simulink model "ModeAdjust"  (R2018b)
settings: Solver=FixedStepDiscrete  StartTime=0.0  StopTime=inf  FixedStep=0.01  RelTol=1e-3
undefined symbols (not defined in the file or in its folder): IfKeSMSbSeatMovBkRclnEnable_Val, IfKeSMSbSeatMovFrwdBkwdEnable_Val, IfKeSMSbSeatMovFtrstEnable_Val, IfKeSMSbSeatMovHdrstFrwdBkwdEnable_Val, IfKeSMSbSeatMovHdUpwdDnwdEnable_Val, IfKeSMSbSeatMovLgrstEnable_Val, IfKeSMSbSeatMovLtwdRtwdEnable_Val, IfVeSMSeStNumConfig, KeSMSbArmscreenMovEnable_Val, KeSMSbSeatMovLgrstExpdEnable_Val, KeSMSuFirstRwStBackPosDelta_Val, KeSMSuFirstRwStBackPosTolr_Val, KeSMSuFirstRwStCushFrntPosDelta_Val, KeSMSuFirstRwStCushFrntPosTolr_Val, KeSMSuFirstRwStCushRePosDelta_Val, KeSMSuFirstRwStCushRePosTolr_Val, KeSMSuFirstRwStFootrestPosDelta_Val, KeSMSuFirstRwStFootrestPosTolr_Val, KeSMSuFirstRwStFwdBkwdPosDelta_Val, KeSMSuFirstRwStFwdBkwdPosTolr_Val, KeSMSuMdMotFinshdTm_Val, KeSMSuMdRetryTm1_Val, KeSMSuModeReqDurgTm_Val, KeSMSuSecRwStArmTochPosDelta_Val, KeSMSuSecRwStArmTochPosTolr_Val, KeSMSuSecRwStBackPosDelta_Val, KeSMSuSecRwStBackPosTolr_Val, KeSMSuSecRwStFtrstUpwdDnwdPosDelta_Val, KeSMSuSecRwStFtrstUpwdDnwdPosTolr_Val, KeSMSuSecRwStFwdBkwdPosDelta_Val, KeSMSuSecRwStFwdBkwdPosTolr_Val, KeSMSuSecRwStHeadrestFwdBkwdPosDelta_Val, KeSMSuSecRwStHeadrestFwdBkwdPosTolr_Val, KeSMSuSecRwStHeadrestUpwdDwnwdPosDelta_Val, KeSMSuSecRwStHeadrestUpwdDwnwdPosTolr_Val, KeSMSuSecRwStLegrestInOutPosDelta_Val, KeSMSuSecRwStLegrestInOutPosTolr_Val, KeSMSuSecRwStLegrestUpwdDwnwdPosDelta_Val, KeSMSuSecRwStLegrestUpwdDwnwdPosTolr_Val, KeSMSuSecRwStLwdRwdPosDelta_Val, KeSMSuSecRwStLwdRwdPosTolr_Val, KeSMSuSecRwStVIPFtrstRefAngle_Val, KeSMSuThirdRwStFwdBkwdPosDelta_Val, KeSMSuThirdRwStFwdBkwdPosTolr_Val, KeSMSuThrdRwCushFoldPosDelta_Val, KeSMSuThrdRwCushFoldPosTolr_Val, KeSMSuThrdRwStBackPosDelta_Val, KeSMSuThrdRwStBackPosTolr_Val, KeSMSw4SLegrstCloseMdSecRwLtStFtrstUpwdDnwdPos_Val, KeSMSw4SLegrstCloseMdSecRwLtStFtrstUpwdDnwdPosMax_Val, KeSMSw4SLegrstCloseMdSecRwLtStFtrstUpwdDnwdPosMin_Val, KeSMSw4SLegrstCloseMdSecRwLtStLgrstOtwdInwdPos_Val, KeSMSw4SLegrstCloseMdSecRwLtStLgrstOtwdInwdPosMax_Val, KeSMSw4SLegrstCloseMdSecRwLtStLgrstOtwdInwdPosMin_Val, KeSMSw4SLegrstCloseMdSecRwLtStLgrstUpwdDnwdPos_Val, KeSMSw4SLegrstCloseMdSecRwLtStLgrstUpwdDnwdPosMax_Val, KeSMSw4SLegrstCloseMdSecRwLtStLgrstUpwdDnwdPosMin_Val, KeSMSw4SLegrstCloseMdSecRwRtStFtrstUpwdDnwdPos_Val, KeSMSw4SLegrstCloseMdSecRwRtStFtrstUpwdDnwdPosMax_Val, KeSMSw4SLegrstCloseMdSecRwRtStFtrstUpwdDnwdPosMin_Val ... (+1138)
libraries: Lib x401
(part 9 of 35)

== system ModeAdjust/ModeAdjustRunnable_sys/ModeAdjust/LyR ==
  SecRwLtStsPoss : Inport
  SecRwLtStPossV : Inport  Port=2
  SecRwRtStChldLkRsp_L : Inport  Port=3
  Recovery_Mod_Left : Inport  Port=4
  ModeStCalib : Inport  Port=5
  StConfig : Inport  Port=6
  SecRwLtStsPoss4s : Inport  Port=7
  SecRwLtStPossV4s : Inport  Port=8
  StConfig4s : Inport  Port=9
  isRtLyArrivedAtTargetPos : Inport  Port=10
  Calib_Ly4sRAdpt : Inport  Port=11
  Enable : EnablePort  StatesWhenEnabling=reset
  Bus Creator1 : BusCreator  Inputs=2
  Bus Selector : BusSelector  OutputSignals=Calib_Drv,Calib_Pass,Calib_2L,Calib_2R,Calib_3L,Calib_3R,Calib_2L4s,Calib_2R4s
  Bus Selector1 : BusSelector  OutputSignals=DrvStConfig,PassStConfig,SecRwLtStConfig,SecRwRtStConfig,ThdRwLtStConfig,ThdRwRtStConfig
  Bus Selector2 : BusSelector  OutputSignals=SecRwLtStConfig,SecRwRtStConfig
  Bus Selector3 : BusSelector  OutputSignals=IfVeSMSuSecRwRtStBkReclnUpwdDnwdPos_Val_read,IfVeSMSuSecRwRtStFrwdBkwdPos_Val_read,IfVeSMSuSecRwRtStHPassStUpwdDnwdPos_Val_read,IfVeSMSuSecRwRtStLgrstUpwdDnwdPos_Val_read,IfVeSMSuSecRwRtStLtwdRtwdPos_Val_read,SecRwRtStArmScrnPos_Val_read
  Bus Selector4 : BusSelector  OutputSignals=IfVeSMSuSecRwRtStBkReclnUpwdDnwdPosV_Val_read,IfVeSMSuSecRwRtStFrwdBkwdPosV_Val_read,IfVeSMSuSecRwRtStHPassStUpwdDnwdPosV_Val_read,IfVeSMSuSecRwRtStLgrstUpwdDnwdPosV_Val_read,IfVeSMSuSecRwRtStLtwdRtwdPosV_Val_read,SecRwRtStArmScrnPosV_Val_read
  Bus Selector5 : BusSelector  OutputSignals=IfVeSMSuSecRwRtStLgrstOtwdInwdPos_Val_read,IfVeSMSuRrRtStFtUpwdDnwdPos_Val_read,IfVeSMSuSecRwRtStHdrstFrwdBkwdPos_Val_read
  Bus Selector6 : BusSelector  OutputSignals=IfVeSMSuSecRwRtStLgrstOtwdInwdPosV_Val_read,IfVeSMSuRrRtStFtUpwdDnwdPosV_Val_read
  Bus Selector7 : BusSelector  OutputSignals=LyRSecRwRtSt.HdrstFrwdBkwdnwdPos,LyRSecRwRtSt.HdrstUpwdPos
  Chart : Stateflow chart  TreatAsAtomicUnit=on
  Chart1 : Stateflow chart  TreatAsAtomicUnit=on
  Logical Operator1 : Logic  AllPortsSameDT=off  OutDataTypeStr=boolean
  Logical Operator{7..10} (4 alike) : Logic  Operator=OR  AllPortsSameDT=off  OutDataTypeStr=boolean
  Logical Operator2 : Logic  AllPortsSameDT=off  OutDataTypeStr=boolean
  Logical Operator3 : Logic  AllPortsSameDT=off  OutDataTypeStr=boolean
  Logical Operator4 : Logic  Operator=NOT  AllPortsSameDT=off  OutDataTypeStr=boolean
  Logical Operator5 : Logic  Inputs=4  AllPortsSameDT=off  OutDataTypeStr=boolean
  Logical Operator6 : Logic  Inputs=3  AllPortsSameDT=off  OutDataTypeStr=boolean
  PA_KeSMSw4SSecRwRtStLgrstUpwdDnwdOpenPos1_Val : Constant  Value=KeSMSw4SSecRwRtStLgrstUpwdDnwdOpenPos1_Val
  R2Lt : Subsystem
  Relational Operator : RelationalOperator  OutDataTypeStr=boolean  RndMeth=Simplest
  Relational Operator1 : RelationalOperator  Operator=<  OutDataTypeStr=boolean  RndMeth=Simplest
  Relational Operator2 : RelationalOperator  Operator=<  OutDataTypeStr=boolean  RndMeth=Simplest
  Unit Delay1 : UnitDelay  SampleTime=-1
  Unit Delay3 : UnitDelay  SampleTime=-1
  Unit Delay4 : UnitDelay  SampleTime=-1
  VIP_TrigJudg : Lib/VIP_TrigJudg  SystemSampleTime=-1
  R2Lt_TrgtPoss : Outport  VectorParamsAs1DForOutWhenUnconnected=on
  IfVeSMSuSecRwLtStRclCmdSrv_Val_writeRec : Outport  Port=2
  isAcsMdFeedBackNew_LyL : Outport  Port=3
  R2Lt_TrgtPoss_2 : Outport  Port=4  VectorParamsAs1DForOutWhenUnconnected=on
  wires:
  R2Lt/11(R2Lt_TrgtPoss_2) -> R2Lt_TrgtPoss_2/1
  Unit Delay1/1 -> Chart/6(Step2done), [lgrstStep2_Chk]
  Logical Operator3/1 -> [lgrstStep3_Chk], Chart/7(Step3done)
  [OpenPos1] -> Chart/4(openpos1)
  PA_KeSMSw4SSecRwRtStLgrstUpwdDnwdOpenPos1_Val/1 -> [OpenPos1]
  [lgrstStep3_ini] -> Chart/10(Step3_ini)
  [lgrstStep2_ini] -> Chart/9(Step2_ini)
  [lgrstStep1_done] -> Chart/5(Step1done)
  R2Lt/9(lgrstStep2_done) -> [lgrstStep2_done]
  R2Lt/10(lgrstStep3_done) -> [lgrstStep3_done]
  R2Lt/8(lgrstStep1_done) -> [lgrstStep1_done]
  R2Lt/6(lgrstStep2_ini) -> [lgrstStep2_ini]
  R2Lt/7(lgrstStep3_ini) -> [lgrstStep3_ini]
  R2Lt/5(lgrstStep1_ini) -> [lgrstStep1_ini]
  [StepEn_LgrstStep3] -> R2Lt/13(StepEn_LgrstStep3)
  [StepEn_LgrstStep2] -> R2Lt/12(StepEn_LgrstStep2)
  [StepEn_LgrstStep1] -> R2Lt/11(StepEn_LgrstStep1)
  [SecRwLtStLgrstUpwdDnwdPos] -> Chart/3(pos)
  Bus Selector5/2 -> [RrLtStFtUpwdDnwdPos]  "<IfVeSMSuRrRtStFtUpwdDnwdPos_Val_read>"
  Bus Selector5/1 -> [SecRwLtStLgrstOtwdInwdPos]  "<IfVeSMSuSecRwRtStLgrstOtwdInwdPos_Val_read>"
  [PosV4s] -> Bus Selector6/1
  Bus Selector6/2 -> [RrLtStFtUpwdDnwdPosV]  "<IfVeSMSuRrRtStFtUpwdDnwdPosV_Val_read>"
  [Pos4s] -> Bus Selector5/1
  Bus Selector6/1 -> [SecRwLtStLgrstOtwdInwdPosV]  "<IfVeSMSuSecRwRtStLgrstOtwdInwdPosV_Val_read>"
  Bus Selector4/1 -> [SecRwLtStBkReclnUpwdDnwdPosV]  "<IfVeSMSuSecRwRtStBkReclnUpwdDnwdPosV_Val_read>"
  Bus Selector4/3 -> [SecRwLtStHPassStUpwdDnwdPosV]  "<IfVeSMSuSecRwRtStHPassStUpwdDnwdPosV_Val_read>"
  Bus Selector3/5 -> [SecRwLtStLtwdRtwdPos]  "<IfVeSMSuSecRwRtStLtwdRtwdPos_Val_read>"
  [Pos] -> Bus Selector3/1
  Bus Selector3/3 -> [SecRwLtStHPassStUpwdDnwdPos]  "<IfVeSMSuSecRwRtStHPassStUpwdDnwdPos_Val_read>"
  Bus Selector4/4 -> [SecRwLtStLgrstUpwdDnwdPosV]  "<IfVeSMSuSecRwRtStLgrstUpwdDnwdPosV_Val_read>"
  Bus Selector4/2 -> [SecRwLtStFrwdBkwdPosV]  "<IfVeSMSuSecRwRtStFrwdBkwdPosV_Val_read>"
  Bus Selector3/2 -> [SecRwLtStFrwdBkwdPos]  "<IfVeSMSuSecRwRtStFrwdBkwdPos_Val_read>"
  Bus Selector3/1 -> [SecRwLtStBkReclnUpwdDnwdPos]  "<IfVeSMSuSecRwRtStBkReclnUpwdDnwdPos_Val_read>"
  Bus Selector3/4 -> [SecRwLtStLgrstUpwdDnwdPos]  "<IfVeSMSuSecRwRtStLgrstUpwdDnwdPos_Val_read>"
  Bus Selector4/5 -> [SecRwLtStLtwdRtwdPosV]  "<IfVeSMSuSecRwRtStLtwdRtwdPosV_Val_read>"
  Bus Selector3/6 -> [R2LtStArmScrnPos]  "<SecRwRtStArmScrnPos_Val_read>"
  Bus Selector4/6 -> [R2LtStArmScrnPosV]  "<SecRwRtStArmScrnPosV_Val_read>"
  [PosV] -> Bus Selector4/1
  [SecRwRtStConfig4s] -> R2Lt/10(StConfig4s)
  Bus Selector2/2 -> [SecRwRtStConfig4s]  "<SecRwRtStConfig>"
  Bus Selector2/1 -> [SecRwLtStConfig4s]  "<SecRwLtStConfig>"
  StConfig4s/1 -> Bus Selector2/1
  SecRwLtStPossV4s/1 -> R2Lt/9(SecRwLtStPossV4s), [PosV4s]
  SecRwLtStsPoss4s/1 -> R2Lt/8(SecRwLtStsPoss4s), [Pos4s]
  Bus Selector/7 -> [ModeStCalib_2L4s]  "<Calib_2L4s>"
  Bus Selector/8 -> [ModeStCalib_2R4s]  "<Calib_2R4s>"
  [SecRwRtStConfig] -> R2Lt/7(StConfig)
  Bus Selector1/5 -> [ThdRwLtStConfig]  "<ThdRwLtStConfig>"
  Bus Selector1/2 -> [PassStConfig]  "<PassStConfig>"
  StConfig/1 -> Bus Selector1/1
  Bus Selector1/4 -> [SecRwRtStConfig]  "<SecRwRtStConfig>"
  Bus Selector1/3 -> [SecRwLtStConfig]  "<SecRwLtStConfig>"
  Bus Selector1/1 -> [DrvStConfig]  "<DrvStConfig>"
  Bus Selector1/6 -> [ThdRwRtStConfig]  "<ThdRwRtStConfig>"
  [Ly_L_DoneFailed] -> Bus Creator1/2  "isRtLyDoneFailed"
  [Ly_L_DoneOK] -> Bus Creator1/1  "isRtLyDoneOK"
  Bus Creator1/1 -> isAcsMdFeedBackNew_LyL/1
  [Recovery_Mod_Left] -> VIP_TrigJudg/1
  [ModeStCalib_2R4s] -> R2Lt/6(ModeStCalib_2L)
  ModeStCalib/1 -> Bus Selector/1
  Bus Selector/4 -> [ModeStCalib_2R]  "<Calib_2R>"
  Bus Selector/6 -> [ModeStCalib_3R]  "<Calib_3R>"
  Bus Selector/1 -> [ModeStCalib_Drv]  "<Calib_Drv>"
  Bus Selector/3 -> [ModeStCalib_2L]  "<Calib_2L>"
  Bus Selector/5 -> [ModeStCalib_3L]  "<Calib_3L>"
  Bus Selector/2 -> [ModeStCalib_Pass]  "<Calib_Pass>"
  Chart1/1(IfVeSMSuSecRwLtStRclCmdSrv_Val_write) -> IfVeSMSuSecRwLtStRclCmdSrv_Val_writeRec/1  "IfVeSMSuSecRwLtStRclCmdSrv_Val_write"
  Chart1/3(Md_L_DoneFailed) -> [Ly_L_DoneFailed]
  Chart1/2(Md_L_DoneOk) -> [Ly_L_DoneOK]
  [Recv_L_DoneFailed] -> Chart1/4(Md_L_DoneFailedRaw)
  [Recv_L_DoneOK] -> Chart1/3(Md_L_DoneOkRaw)
  [R2LtST_BkHd_done] -> Chart/2(R2Lt_done)
  [R2LtST_BkHd_ini] -> Chart/1(R2Lt_ini)
  R2Lt/2(R2Lt_BkHd_done) -> [R2LtST_BkHd_done]
  SecRwRtStChldLkRsp_L/1 -> R2Lt/5(SecRwRtStChldLkRsp_L)
  SecRwLtStPossV/1 -> R2Lt/4(SecRwLtStPossV), [PosV]
  SecRwLtStsPoss/1 -> R2Lt/3(SecRwLtStsPoss), [Pos]
  R2Lt/3(R2Lt_TrgtPoss) -> R2Lt_TrgtPoss/1
  [EZE_TrigL] -> R2Lt/1(Mode_Trig)
  VIP_TrigJudg/1 -> [EZE_TrigL]
  [Step1_En] -> R2Lt/2(Step1En)
  R2Lt/1(R2Lt_BkHd_Ini) -> [R2LtST_BkHd_ini]
  Recovery_Mod_Left/1 -> [Recovery_Mod_Left]
  [IfVeSMSuSecRwLtStRclCmdSrv_Val_writeRaw] -> Chart1/2(IfVeSMSuSecRwLtStRclCmdSrv_Val_writeRaw)
  R2Lt/4(IfVeSMSuSecRwLtStRclCmdSrv_Val_writeRaw) -> [IfVeSMSuSecRwLtStRclCmdSrv_Val_writeRaw]
  [OpenPos1] -> Relational Operator/2
  [lgrstStep2_Chk] -> Unit Delay4/1
  Unit Delay3/1 -> Logical Operator2/1
  [lgrstStep3_done] -> Logical Operator3/1
  [SecRwLtStLgrstUpwdDnwdPos] -> Relational Operator/1
  Logical Operator2/1 -> Unit Delay1/1
  [lgrstStep2_done] -> Logical Operator2/2
  Relational Operator/1 -> Unit Delay3/1
  Unit Delay4/1 -> Logical Operator3/2
  Logical Operator4/1 -> [Recv_L_DoneFailed]
  isRtLyArrivedAtTargetPos/1 -> [Recv_L_DoneOK], Logical Operator4/1
  [HdUp_Done] -> Logical Operator5/3
  [HFwd_Done] -> Logical Operator5/4
  [failflg] -> Logical Operator7/2
  Logical Operator6/1 -> Logical Operator7/1
  [R2LtST_BkHd_done] -> Logical Operator5/2
  Logical Operator5/1 -> Chart1/1(Left_Done)
  Logical Operator7/1 -> Logical Operator5/1
  Chart/1(R2Lt_En) -> [Step1_En]
  Chart/7(failflg) -> [failflg]
  Chart/5(HdUp_En) -> [HdUp_En]
  Chart/2(StepEn_LgrstStep1) -> [StepEn_LgrstStep1]
  Bus Selector7/1 -> Relational Operator1/2  "<HdrstFrwdBkwdnwdPos>"
  [SecRwLtStHdrstFrwdBkwdPos] -> Relational Operator1/1
  Logical Operator1/1 -> Chart/11(chkhdflg)
  Chart/6(HdFwd_En) -> [HdFwd_En]
  Relational Operator1/1 -> Logical Operator1/1
  [ModeStCalib_2R4s] -> Bus Selector7/1
  [SecRwLtStHPassStUpwdDnwdPos] -> Relational Operator2/1
  Bus Selector7/2 -> Relational Operator2/2  "<HdrstUpwdPos>"
  Chart/4(StepEn_LgrstStep3) -> [StepEn_LgrstStep3]
  Relational Operator2/1 -> Logical Operator1/2
  Chart/3(StepEn_LgrstStep2) -> [StepEn_LgrstStep2]
  [HdUp_En] -> R2Lt/14(HdUp_En)
  [HdFwd_En] -> R2Lt/15(HdFwd_En)
  R2Lt/14(R2Lt_HdFwd_Ini) -> [HFwd_ini]
  R2Lt/13(R2Lt_HdUp_Done) -> [HdUp_Done]
  R2Lt/15(R2Lt_HdFwd_Done) -> [HFwd_Done]
  R2Lt/12(R2Lt_HdUp_Ini) -> [HdUp_ini]
  Bus Selector5/3 -> [SecRwLtStHdrstFrwdBkwdPos]  "<IfVeSMSuSecRwRtStHdrstFrwdBkwdPos_Val_read>"
  [lgrstStep1_done] -> Logical Operator8/1
  [lgrstStep1_ini] -> Logical Operator8/2
  Logical Operator8/1 -> Logical Operator6/1
  Logical Operator9/1 -> Logical Operator6/2
  [lgrstStep2_Chk] -> Logical Operator9/1
  [lgrstStep2_ini] -> Logical Operator9/2
  Logical Operator10/1 -> Logical Operator6/3
  [lgrstStep3_Chk] -> Logical Operator10/1
  [lgrstStep3_ini] -> Logical Operator10/2
  [HdUp_ini] -> Chart/14(HdUp_ini)
  [HFwd_ini] -> Chart/15(HdFwd_ini)
  Calib_Ly4sRAdpt/1 -> R2Lt/16(Calib_Ly4sRAdpt)
  [lgrstStep1_ini] -> Chart/8(Step1_ini)
  [HdUp_Done] -> Chart/12(HdUp_Done)
  [HFwd_Done] -> Chart/13(HdFwd_Done)

== system ModeAdjust/ModeAdjustRunnable_sys/ModeAdjust/ModeEnChek ==
  modestate32 : Inport
  Chart3 : Stateflow chart  TreatAsAtomicUnit=on
  Demux : Demux  Outputs=32
  Terminator_{6..17} (12 alike) : Terminator
  VIP_L_En : Outport
  VIP_R_En : Outport  Port=2
  Recovery_L_En : Outport  Port=3
  Recovery_R_En : Outport  Port=4
  Lug_L_En : Outport  Port=5
  Lug_R_En : Outport  Port=6
  EZE_En : Outport  Port=7
  EZQ_En : Outport  Port=8
  VIPAll_En : Outport  Port=9
  LugAll_En : Outport  Port=10
  INTM_En : Outport  Port=11
  FAMLY_L_En : Outport  Port=12
  FAMLY_R_En : Outport  Port=13
  LyL_En : Outport  Port=14
  LyR_En : Outport  Port=15
  LgrstOpenL_En : Outport  Port=16
  LgrstCloseL_En : Outport  Port=17
  LgrstOpenR_En : Outport  Port=18
  LgrstCloseR_En : Outport  Port=19
  INTMR_En : Outport  Port=20
  wires:
  Chart3/1(ModeArray) -> Demux/1
  Demux/1 -> [EZE_En]
  Demux/2 -> [VIPAll_En]
  Demux/3 -> [LugAll_En]
  Demux/4 -> [EZQ_En]
  Demux/5 -> [INTM_En]
  Demux/6 -> [FAMLY_R_En]
  Demux/7 -> [FAMLY_L_En]
  Demux/8 -> [LugL_En]
  Demux/9 -> [LugR_En]
  Demux/10 -> [VIPL_En]
  Demux/12 -> [VIPR_En]
  Demux/11 -> [RecoveryL_En]
  Demux/13 -> [RecoveryR_En]
  Demux/14 -> [LyL_En]
  Demux/15 -> [LyR_En]
  modestate32/1 -> [modestate32], Chart3/1(ModeState32)
  [EZE_En] -> EZE_En/1
  [EZQ_En] -> EZQ_En/1
  [VIPL_En] -> VIP_L_En/1
  [VIPR_En] -> VIP_R_En/1
  [RecoveryL_En] -> Recovery_L_En/1
  [RecoveryR_En] -> Recovery_R_En/1
  [LugL_En] -> Lug_L_En/1
  [LugR_En] -> Lug_R_En/1
  [VIPAll_En] -> VIPAll_En/1
  [LugAll_En] -> LugAll_En/1
  Demux/16 -> [LgrstOpenL_En]
  Demux/17 -> [LgrstCloseL_En]
  Demux/18 -> [LgrstOpenR_En]
  Demux/19 -> [LgrstCloseR_En]
  Demux/20 -> [INTMR_En]
  Demux/21 -> Terminator_6/1
  Demux/22 -> Terminator_7/1
  Demux/23 -> Terminator_8/1
  Demux/24 -> Terminator_9/1
  Demux/25 -> Terminator_10/1
  Demux/26 -> Terminator_11/1
  Demux/27 -> Terminator_12/1
  Demux/28 -> Terminator_13/1
  Demux/29 -> Terminator_14/1
  Demux/30 -> Terminator_15/1
  Demux/31 -> Terminator_16/1
  Demux/32 -> Terminator_17/1
  [INTM_En] -> INTM_En/1
  [FAMLY_L_En] -> FAMLY_L_En/1
  [FAMLY_R_En] -> FAMLY_R_En/1
  [LyR_En] -> LyR_En/1
  [LyL_En] -> LyL_En/1
  [LgrstOpenL_En] -> LgrstOpenL_En/1
  [LgrstCloseL_En] -> LgrstCloseL_En/1
  [LgrstOpenR_En] -> LgrstOpenR_En/1
  [LgrstCloseR_En] -> LgrstCloseR_En/1
  [INTMR_En] -> INTMR_En/1

== system ModeAdjust/ModeAdjustRunnable_sys/ModeAdjust/PassFailFeedBack ==
  FeedBackNew_EZE : Inport
  EZE_En : Inport  Port=2
  FeedBack_Def : Inport  Port=3
  FeedBackNew_EZQ : Inport  Port=4
  EZQ_En : Inport  Port=5
  FeedBackNEW_VIPL : Inport  Port=6
  VIP_L : Inport  Port=7
  FeedBackNEW_VIPR : Inport  Port=8
  VIP_R : Inport  Port=9
  FeedBackNew_LugL : Inport  Port=10
  Lug_L : Inport  Port=11
  FeedBackNew_LugR : Inport  Port=12
  Lug_R : Inport  Port=13
  FeedBackNew_RevL : Inport  Port=14
  Recovery_L : Inport  Port=15
  FeedBackNew_RevR : Inport  Port=16
  Recovery_R : Inport  Port=17
  FeedBackNew_INTM : Inport  Port=18
  INTM_En : Inport  Port=19
  FeedBackNEW_FAMLYL : Inport  Port=20
  FAMLY_L_En : Inport  Port=21
  FeedBackNEW_FAMLYR : Inport  Port=22
  FAMLY_R_En : Inport  Port=23
  FeedBackNew_LyL : Inport  Port=24
  LyL_En : Inport  Port=25
  FeedBackNew_LyR : Inport  Port=26
  LyR_En : Inport  Port=27
  FeedBackNew_INTMR : Inport  Port=28
  INTMR_En : Inport  Port=29
  FeedBackNew_LgrstOpenL : Inport  Port=30
  LgrstOpenL_En : Inport  Port=31
  FeedBackNew_LgrstOpenR : Inport  Port=32
  LgrstOpenR_En : Inport  Port=33
  FeedBackNew_LgrstCloseL : Inport  Port=34
  LgrstCloseL_En : Inport  Port=35
  FeedBackNew_LgrstCloseR : Inport  Port=36
  LgrstCloseR_En : Inport  Port=37
  Bus Creator{1..10,12..19} (18 alike) : BusCreator  Inputs=2
  Bus Selector1 : BusSelector  OutputSignals=isINTMDoneOK,isINTMDoneFailed
  Bus Selector10 : BusSelector  OutputSignals=isAcsMdExtDoneOK,isAcsMdExtDoneFailed
  Bus Selector11 : BusSelector  OutputSignals=isLfVipDoneOK,isLfVipDoneFailed
  Bus Selector12 : BusSelector  OutputSignals=isRtVipDoneOK,isRtVipDoneFailed
  Bus Selector13 : BusSelector  OutputSignals=isRtVipDoneOK,isRtVipDoneFailed
  Bus Selector14 : BusSelector  OutputSignals=isLfLugDoneOK,isLfLugDoneFailed
  Bus Selector15 : BusSelector  OutputSignals=isLfLugDoneOK,isLfLugDoneFailed
  Bus Selector16 : BusSelector  OutputSignals=isRtLugDoneOK,isRtLugDoneFailed
  Bus Selector17 : BusSelector  OutputSignals=isLfRecoveryDoneOK,isLfRecoveryDoneFailed
  Bus Selector18 : BusSelector  OutputSignals=isRfRecoveryDoneOK,isRfRecoveryDoneFailed
  Bus Selector19 : BusSelector  OutputSignals=isRtLugDoneOK,isRtLugDoneFailed
  Bus Selector2 : BusSelector  OutputSignals=isINTMDoneOK,isINTMDoneFailed
  Bus Selector20 : BusSelector  OutputSignals=isLfRecoveryDoneOK,isLfRecoveryDoneFailed
  Bus Selector21 : BusSelector  OutputSignals=isRfRecoveryDoneOK,isRfRecoveryDoneFailed
  Bus Selector22 : BusSelector  OutputSignals=isRtFamlyDoneOK,isRtFamlyDoneFailed
  Bus Selector23 : BusSelector  OutputSignals=isLfLyDoneOK,isLfLyDoneFailed
  Bus Selector24 : BusSelector  OutputSignals=isLfLyDoneOK,isLfLyDoneFailed
  Bus Selector25 : BusSelector  OutputSignals=isRtLyDoneOK,isRtLyDoneFailed
  Bus Selector26 : BusSelector  OutputSignals=isRtLyDoneOK,isRtLyDoneFailed
  Bus Selector27 : BusSelector  OutputSignals=isINTMRDoneOK,isINTMRDoneFailed
  Bus Selector28 : BusSelector  OutputSignals=isINTMRDoneOK,isINTMRDoneFailed
  Bus Selector29 : BusSelector  OutputSignals=isLgrstOpenLDoneOK,isLgrstOpenLDoneFailed
  Bus Selector3 : BusSelector  OutputSignals=isLfFamlyDoneOK,isLfFamlyDoneFailed
  Bus Selector30 : BusSelector  OutputSignals=isLgrstOpenLDoneOK,isLgrstOpenLDoneFailed
  Bus Selector31 : BusSelector  OutputSignals=isLgrstOpenRDoneOK,isLgrstOpenRDoneFailed
  Bus Selector32 : BusSelector  OutputSignals=isLgrstOpenRDoneOK,isLgrstOpenRDoneFailed
  Bus Selector33 : BusSelector  OutputSignals=isLgrstCloseLDoneOK,isLgrstCloseLDoneFailed
  Bus Selector34 : BusSelector  OutputSignals=isLgrstCloseLDoneOK,isLgrstCloseLDoneFailed
  Bus Selector35 : BusSelector  OutputSignals=isLgrstCloseRDoneOK,isLgrstCloseRDoneFailed
  Bus Selector36 : BusSelector  OutputSignals=isLgrstCloseRDoneOK,isLgrstCloseRDoneFailed
  Bus Selector4 : BusSelector  OutputSignals=isLfFamlyDoneOK,isLfFamlyDoneFailed
  Bus Selector5 : BusSelector  OutputSignals=isRtFamlyDoneOK,isRtFamlyDoneFailed
  Bus Selector6 : BusSelector  OutputSignals=isLfVipDoneOK,isLfVipDoneFailed
  Bus Selector7 : BusSelector  OutputSignals=isAcsMdEntryDoneOK,isAcsMdEntryDoneFailed
  Bus Selector8 : BusSelector  OutputSignals=isAcsMdEntryDoneOK,isAcsMdEntryDoneFailed
  Bus Selector9 : BusSelector  OutputSignals=isAcsMdExtDoneOK,isAcsMdExtDoneFailed
  Switch{,1..17} (18 alike) : Switch  Criteria=u2 > Threshold
  <isAcsMdEntryDoneOK> : Outport
  <isAcsMdEntryDoneFailed> : Outport  Port=2
  <isAcsMdExtDoneOK> : Outport  Port=3
  <isAcsMdExtDoneFailed> : Outport  Port=4
  <isLfVipDoneOK> : Outport  Port=5
  <isLfVipDoneFailed> : Outport  Port=6
  <isRtVipDoneOK> : Outport  Port=7
  <isRtVipDoneFailed> : Outport  Port=8
  <isLfLugDoneOK> : Outport  Port=9
  <isLfLugDoneFailed> : Outport  Port=10
  <isRtLugDoneOK> : Outport  Port=11
  <isRtLugDoneFailed> : Outport  Port=12
  <isLfRecoveryDoneOK> : Outport  Port=13
  <isLfRecoveryDoneFailed> : Outport  Port=14
  <isRfRecoveryDoneOK> : Outport  Port=15
  <isRfRecoveryDoneFailed> : Outport  Port=16
  <isINTMDoneOK> : Outport  Port=17
  <isINTMDoneFailed> : Outport  Port=18
  <isLfFamlyOK> : Outport  Port=19
  <isLfFamlyDoneFailed> : Outport  Port=20
  <isRtFamlyDoneOK> : Outport  Port=21
  <isRtFamlyDoneFailed> : Outport  Port=22
  <isLfLyDoneOK> : Outport  Port=23
  <isLfLyDoneFailed> : Outport  Port=24
  <isRtLyDoneOK> : Outport  Port=25
  <isRtLyDoneFailed> : Outport  Port=26
  <isINTMRDoneOK> : Outport  Port=27
  <isINTMRDoneFailed> : Outport  Port=28
  <isLgrstOpenLDoneOK> : Outport  Port=29
  <isLgrstOpenLDoneFailed> : Outport  Port=30
  <isLgrstOpenRDoneOK> : Outport  Port=31
  <isLgrstOpenRDoneFailed> : Outport  Port=32
  <isLgrstCloseLDoneOK> : Outport  Port=33
  <isLgrstCloseLDoneFailed> : Outport  Port=34
  <isLgrstCloseRDoneOK> : Outport  Port=35
  <isLgrstCloseRDoneFailed> : Outport  Port=36
  wires:
  Bus Creator18/1 -> Switch6/3
  Bus Selector13/1 -> <isRtVipDoneOK>/1  "<isRtVipDoneOK>"
  [FeedBack_Def] -> Bus Selector19/1
  Bus Selector17/2 -> <isLfRecoveryDoneFailed>/1  "<isLfRecoveryDoneFailed>"
  Bus Selector21/1 -> Bus Creator19/1  "<isRfRecoveryDoneOK>"
  Bus Selector16/2 -> <isRtLugDoneFailed>/1  "<isRtLugDoneFailed>"
  Switch7/1 -> Bus Selector18/1
  [FeedBack_Def] -> Bus Selector20/1
  Bus Selector7/2 -> <isAcsMdEntryDoneFailed>/1  "<isAcsMdEntryDoneFailed>"
  Bus Selector19/2 -> Bus Creator17/2  "<isRtLugDoneFailed>"
  Bus Selector11/1 -> <isLfVipDoneOK>/1  "<isLfVipDoneOK>"
  Lug_R/1 -> Switch5/2
  Bus Selector10/1 -> <isAcsMdExtDoneOK>/1  "<isAcsMdExtDoneOK>"
  Bus Selector21/2 -> Bus Creator19/2  "<isRfRecoveryDoneFailed>"
  Bus Selector20/1 -> Bus Creator18/1  "<isLfRecoveryDoneOK>"
  Bus Creator12/1 -> Switch/3
  Bus Selector20/2 -> Bus Creator18/2  "<isLfRecoveryDoneFailed>"
  Bus Creator15/1 -> Switch3/3
  Bus Selector8/2 -> Bus Creator12/2  "<isAcsMdEntryDoneFailed>"
  Bus Selector14/1 -> Bus Creator16/1  "<isLfLugDoneOK>"
  Bus Selector18/2 -> <isRfRecoveryDoneFailed>/1  "<isRfRecoveryDoneFailed>"
  Bus Selector6/1 -> Bus Creator14/1  "<isLfVipDoneOK>"
  Switch5/1 -> Bus Selector16/1
  Bus Selector6/2 -> Bus Creator14/2  "<isLfVipDoneFailed>"
  Bus Creator13/1 -> Switch1/3
  Bus Selector9/1 -> Bus Creator13/1  "<isAcsMdExtDoneOK>"
  Switch1/1 -> Bus Selector10/1
  FeedBack_Def/1 -> [FeedBack_Def], Bus Selector8/1
  Bus Selector14/2 -> Bus Creator16/2  "<isLfLugDoneFailed>"
  Switch6/1 -> Bus Selector17/1
  EZQ_En/1 -> Switch1/2
  Bus Selector19/1 -> Bus Creator17/1  "<isRtLugDoneOK>"
  Bus Selector7/1 -> <isAcsMdEntryDoneOK>/1  "<isAcsMdEntryDoneOK>"
  Switch3/1 -> Bus Selector13/1
  Bus Selector17/1 -> <isLfRecoveryDoneOK>/1  "<isLfRecoveryDoneOK>"
  Bus Selector12/1 -> Bus Creator15/1  "<isRtVipDoneOK>"
  Bus Selector8/1 -> Bus Creator12/1  "<isAcsMdEntryDoneOK>"
  Bus Selector18/1 -> <isRfRecoveryDoneOK>/1  "<isRfRecoveryDoneOK>"
  Bus Selector15/1 -> <isLfLugDoneOK>/1  "<isLfLugDoneOK>"
  Bus Selector12/2 -> Bus Creator15/2  "<isRtVipDoneFailed>"
  Switch4/1 -> Bus Selector15/1
  [FeedBack_Def] -> Bus Selector14/1
  FeedBackNew_RevR/1 -> Switch7/1
  [FeedBack_Def] -> Bus Selector12/1
  Bus Selector13/2 -> <isRtVipDoneFailed>/1  "<isRtVipDoneFailed>"
  FeedBackNew_EZE/1 -> Switch/1
  Bus Selector9/2 -> Bus Creator13/2  "<isAcsMdExtDoneFailed>"
  EZE_En/1 -> Switch/2
  [FeedBack_Def] -> Bus Selector9/1
  Bus Selector15/2 -> <isLfLugDoneFailed>/1  "<isLfLugDoneFailed>"
  Switch/1 -> Bus Selector7/1
  Switch2/1 -> Bus Selector11/1
  Bus Creator16/1 -> Switch4/3
  [FeedBack_Def] -> Bus Selector21/1
  VIP_R/1 -> Switch3/2
  Bus Creator19/1 -> Switch7/3
  Bus Creator17/1 -> Switch5/3
  Bus Selector11/2 -> <isLfVipDoneFailed>/1  "<isLfVipDoneFailed>"
  Bus Selector10/2 -> <isAcsMdExtDoneFailed>/1  "<isAcsMdExtDoneFailed>"
  FeedBackNew_RevL/1 -> Switch6/1
  Recovery_L/1 -> Switch6/2
  VIP_L/1 -> Switch2/2
  Recovery_R/1 -> Switch7/2
  Bus Selector16/1 -> <isRtLugDoneOK>/1  "<isRtLugDoneOK>"
  Lug_L/1 -> Switch4/2
  FeedBackNew_EZQ/1 -> Switch1/1
  [FeedBack_Def] -> Bus Selector6/1
  Bus Creator14/1 -> Switch2/3
  FeedBackNEW_VIPL/1 -> Switch2/1
  FeedBackNEW_VIPR/1 -> Switch3/1
  FeedBackNew_LugL/1 -> Switch4/1
  FeedBackNew_LugR/1 -> Switch5/1
  INTM_En/1 -> Switch8/2
  FeedBackNew_INTM/1 -> Switch8/1
  Bus Selector1/1 -> <isINTMDoneOK>/1  "<isINTMDoneOK>"
  Switch8/1 -> Bus Selector1/1
  Bus Selector2/2 -> Bus Creator1/2  "<isINTMDoneFailed>"
  Bus Selector2/1 -> Bus Creator1/1  "<isINTMDoneOK>"
  [FeedBack_Def] -> Bus Selector2/1
  Bus Selector1/2 -> <isINTMDoneFailed>/1  "<isINTMDoneFailed>"
  Bus Creator1/1 -> Switch8/3
  Bus Creator2/1 -> Switch9/3
  Bus Selector3/2 -> <isLfFamlyDoneFailed>/1  "<isLfFamlyDoneFailed>"
  [FeedBack_Def] -> Bus Selector4/1
  Bus Selector4/1 -> Bus Creator2/1  "<isLfFamlyDoneOK>"
  Bus Selector4/2 -> Bus Creator2/2  "<isLfFamlyDoneFailed>"
  Switch9/1 -> Bus Selector3/1
  Bus Selector3/1 -> <isLfFamlyOK>/1  "<isLfFamlyDoneOK>"
  FeedBackNEW_FAMLYL/1 -> Switch9/1
  FAMLY_L_En/1 -> Switch9/2
  FAMLY_R_En/1 -> Switch10/2
  FeedBackNEW_FAMLYR/1 -> Switch10/1
  Bus Selector5/1 -> <isRtFamlyDoneOK>/1  "<isRtFamlyDoneOK>"
  Switch10/1 -> Bus Selector5/1
  Bus Selector22/2 -> Bus Creator3/2  "<isRtFamlyDoneFailed>"
  Bus Selector22/1 -> Bus Creator3/1  "<isRtFamlyDoneOK>"
  [FeedBack_Def] -> Bus Selector22/1
  Bus Selector5/2 -> <isRtFamlyDoneFailed>/1  "<isRtFamlyDoneFailed>"
  Bus Creator3/1 -> Switch10/3
  Bus Creator4/1 -> Switch11/3
  Bus Selector24/2 -> <isLfLyDoneFailed>/1  "<isLfLyDoneFailed>"
  [FeedBack_Def] -> Bus Selector23/1
  Bus Selector23/1 -> Bus Creator4/1  "<isLfLyDoneOK>"
  Bus Selector23/2 -> Bus Creator4/2  "<isLfLyDoneFailed>"
  Switch11/1 -> Bus Selector24/1
  Bus Selector24/1 -> <isLfLyDoneOK>/1  "<isLfLyDoneOK>"
  FeedBackNew_LyL/1 -> Switch11/1
  LyL_En/1 -> Switch11/2
  LyR_En/1 -> Switch12/2
  FeedBackNew_LyR/1 -> Switch12/1
  Bus Selector26/1 -> <isRtLyDoneOK>/1  "<isRtLyDoneOK>"
  Switch12/1 -> Bus Selector26/1
  Bus Selector25/2 -> Bus Creator5/2  "<isRtLyDoneFailed>"
  Bus Selector25/1 -> Bus Creator5/1  "<isRtLyDoneOK>"
  [FeedBack_Def] -> Bus Selector25/1
  Bus Selector26/2 -> <isRtLyDoneFailed>/1  "<isRtLyDoneFailed>"
  Bus Creator5/1 -> Switch12/3
  Bus Creator6/1 -> Switch13/3
  Bus Selector28/2 -> <isINTMRDoneFailed>/1  "<isINTMRDoneFailed>"
  [FeedBack_Def] -> Bus Selector27/1
  Bus Selector27/1 -> Bus Creator6/1  "<isINTMRDoneOK>"
  Bus Selector27/2 -> Bus Creator6/2  "<isINTMRDoneFailed>"
  Switch13/1 -> Bus Selector28/1
  Bus Selector28/1 -> <isINTMRDoneOK>/1  "<isINTMRDoneOK>"
  FeedBackNew_INTMR/1 -> Switch13/1
  INTMR_En/1 -> Switch13/2
  LgrstOpenL_En/1 -> Switch14/2
  FeedBackNew_LgrstOpenL/1 -> Switch14/1
  Bus Selector30/1 -> <isLgrstOpenLDoneOK>/1  "<isLgrstOpenLDoneOK>"
  Switch14/1 -> Bus Selector30/1
  Bus Selector29/2 -> Bus Creator7/2  "<isLgrstOpenLDoneFailed>"
  Bus Selector29/1 -> Bus Creator7/1  "<isLgrstOpenLDoneOK>"
  [FeedBack_Def] -> Bus Selector29/1
  Bus Selector30/2 -> <isLgrstOpenLDoneFailed>/1  "<isLgrstOpenLDoneFailed>"
  Bus Creator7/1 -> Switch14/3
  Bus Creator8/1 -> Switch15/3
  Bus Selector32/2 -> <isLgrstOpenRDoneFailed>/1  "<isLgrstOpenRDoneFailed>"
  [FeedBack_Def] -> Bus Selector31/1
  Bus Selector31/1 -> Bus Creator8/1  "<isLgrstOpenRDoneOK>"
  Bus Selector31/2 -> Bus Creator8/2  "<isLgrstOpenRDoneFailed>"
  Switch15/1 -> Bus Selector32/1
  Bus Selector32/1 -> <isLgrstOpenRDoneOK>/1  "<isLgrstOpenRDoneOK>"
  FeedBackNew_LgrstOpenR/1 -> Switch15/1
  LgrstOpenR_En/1 -> Switch15/2
  LgrstCloseL_En/1 -> Switch16/2
  FeedBackNew_LgrstCloseL/1 -> Switch16/1
  Bus Selector34/1 -> <isLgrstCloseLDoneOK>/1  "<isLgrstCloseLDoneOK>"
  Switch16/1 -> Bus Selector34/1
  Bus Selector33/2 -> Bus Creator9/2  "<isLgrstCloseLDoneFailed>"
  Bus Selector33/1 -> Bus Creator9/1  "<isLgrstCloseLDoneOK>"
  [FeedBack_Def] -> Bus Selector33/1
  Bus Selector34/2 -> <isLgrstCloseLDoneFailed>/1  "<isLgrstCloseLDoneFailed>"
  Bus Creator9/1 -> Switch16/3
  Bus Creator10/1 -> Switch17/3
  Bus Selector36/2 -> <isLgrstCloseRDoneFailed>/1  "<isLgrstCloseRDoneFailed>"
  [FeedBack_Def] -> Bus Selector35/1
  Bus Selector35/1 -> Bus Creator10/1  "<isLgrstCloseRDoneOK>"
  Bus Selector35/2 -> Bus Creator10/2  "<isLgrstCloseRDoneFailed>"
  Switch17/1 -> Bus Selector36/1
  Bus Selector36/1 -> <isLgrstCloseRDoneOK>/1  "<isLgrstCloseRDoneOK>"
  FeedBackNew_LgrstCloseR/1 -> Switch17/1
  LgrstCloseR_En/1 -> Switch17/2

== system ModeAdjust/ModeAdjustRunnable_sys/ModeAdjust/RecoveryL ==
  SecRwLtStsPoss : Inport
  SecRwLtStPossV : Inport  Port=2
  SecRwRtStChldLkRsp_L : Inport  Port=3
  Recovery_Mod_Left : Inport  Port=4
  ModeStCalib : Inport  Port=5
  StConfig : Inport  Port=6
  DrvCurPos : Inport  Port=7
  DrvCurPosV : Inport  Port=8
  isLfRecoveryArrivedAtTargetPos : Inport  Port=9
  Enable : EnablePort  StatesWhenEnabling=reset
  Bus Creator1 : BusCreator  Inputs=2
  Bus Selector : BusSelector  OutputSignals=Calib_Drv,Calib_Pass,Calib_2L,Calib_2R,Calib_3L,Calib_3R
  Bus Selector1 : BusSelector  OutputSignals=DrvStConfig,PassStConfig,SecRwLtStConfig,SecRwRtStConfig,ThdRwLtStConfig,ThdRwRtStConfig
  Chart : Stateflow chart  TreatAsAtomicUnit=on
  Chart1 : Stateflow chart  TreatAsAtomicUnit=on
  Drv : Subsystem
  Logical Operator2 : Logic  AllPortsSameDT=off  OutDataTypeStr=boolean
  Logical Operator3 : Logic  Operator=NOT  AllPortsSameDT=off  OutDataTypeStr=boolean
  R2Lt : Subsystem
  VIP_TrigJudg : Lib/VIP_TrigJudg  SystemSampleTime=-1
  R2Lt_TrgtPoss : Outport  VectorParamsAs1DForOutWhenUnconnected=on
  IfVeSMSuSecRwLtStRclCmdSrv_Val_writeRec : Outport  Port=2
  isAcsMdFeedBackNew_RecoveryL : Outport  Port=3
  RecoveryLDone : Outport  Port=4
  DrvStTrgtPoss : Outport  Port=5  VectorParamsAs1DForOutWhenUnconnected=on
  IfVeSMSbDrvStRclCmdSrv_Val_write : Outport  Port=6
  wires:
  R2Lt/4(IfVeSMSuSecRwLtStRclCmdSrv_Val_writeRaw) -> [IfVeSMSuSecRwLtStRclCmdSrv_Val_writeRaw]
  [IfVeSMSuSecRwLtStRclCmdSrv_Val_writeRaw] -> Chart1/2(IfVeSMSuSecRwLtStRclCmdSrv_Val_writeRaw)
  Recovery_Mod_Left/1 -> [Recovery_Mod_Left]
  R2Lt/1(R2Lt_Recovery_Ini) -> [R2LtST_Recovery_ini]
  [L_R2Lt_En] -> R2Lt/2(Step1En)
  VIP_TrigJudg/1 -> [EZE_TrigL]
  [EZE_TrigL] -> R2Lt/1(Mode_Trig)
  R2Lt/3(R2Lt_TrgtPoss) -> R2Lt_TrgtPoss/1
  SecRwLtStsPoss/1 -> R2Lt/3(SecRwLtStsPoss)
  SecRwLtStPossV/1 -> R2Lt/4(SecRwLtStPossV)
  SecRwRtStChldLkRsp_L/1 -> Drv/7(SecRwRtStChldLkRsp_L), R2Lt/5(SecRwRtStChldLkRsp_L)
  R2Lt/2(R2Lt_Recovery_done) -> [R2LtST_Recovery_done]
  [R2LtST_Recovery_ini] -> Chart/1(R2Lt_ini)
  [R2LtST_Recovery_done] -> Chart/2(R2Lt_done)
  Chart/1(R2Lt_En) -> [L_R2Lt_En]
  [Recv_L_DoneOK] -> Chart1/3(Md_L_DoneOkRaw)
  [Recv_L_DoneFailed] -> Chart1/4(Md_L_DoneFailedRaw)
  Chart1/2(Md_L_DoneOk) -> [Recovery_L_DoneOK]
  Chart1/3(Md_L_DoneFailed) -> [Recovery_L_DoneFailed]
  Chart1/1(IfVeSMSuSecRwLtStRclCmdSrv_Val_write) -> IfVeSMSuSecRwLtStRclCmdSrv_Val_writeRec/1  "IfVeSMSuSecRwLtStRclCmdSrv_Val_write"
  Bus Selector/2 -> [ModeStCalib_Pass]  "<Calib_Pass>"
  Bus Selector/5 -> [ModeStCalib_3L]  "<Calib_3L>"
  Bus Selector/3 -> [ModeStCalib_2L]  "<Calib_2L>"
  Bus Selector/1 -> [ModeStCalib_Drv]  "<Calib_Drv>"
  Bus Selector/6 -> [ModeStCalib_3R]  "<Calib_3R>"
  Bus Selector/4 -> [ModeStCalib_2R]  "<Calib_2R>"
  ModeStCalib/1 -> Bus Selector/1
  [ModeStCalib_2L] -> R2Lt/6(ModeStCalib_2L)
  [Recovery_Mod_Left] -> VIP_TrigJudg/1
  Bus Creator1/1 -> isAcsMdFeedBackNew_RecoveryL/1
  [Recovery_L_DoneOK] -> Bus Creator1/1  "isLfRecoveryDoneOK"
  [Recovery_L_DoneFailed] -> Bus Creator1/2  "isLfRecoveryDoneFailed"
  Bus Selector1/6 -> [ThdRwRtStConfig]  "<ThdRwRtStConfig>"
  Bus Selector1/1 -> [DrvStConfig]  "<DrvStConfig>"
  Bus Selector1/3 -> [SecRwLtStConfig]  "<SecRwLtStConfig>"
  Bus Selector1/4 -> [SecRwRtStConfig]  "<SecRwRtStConfig>"
  StConfig/1 -> Bus Selector1/1
  Bus Selector1/2 -> [PassStConfig]  "<PassStConfig>"
  Bus Selector1/5 -> [ThdRwLtStConfig]  "<ThdRwLtStConfig>"
  [SecRwLtStConfig] -> R2Lt/7(StConfig)
  DrvCurPosV/1 -> Drv/4(DrvCurPosV)
  [DrvStConfig] -> Drv/6(StConfig)
  Drv/1(DrvSt_Step1_ini) -> [DrvST_Step1_ini]
  [ModeStCalib_Drv] -> Drv/5(ModeStCalib_Drv)
  [EZE_TrigL] -> Drv/1(Mode_Trig)
  Drv/2(DrvSt_Step1_done) -> [DrvST_Step1_done]
  DrvCurPos/1 -> Drv/3(DrvCurPos)
  Drv/3(Recv_DrvStTrgtPoss) -> DrvStTrgtPoss/1
  [DrvST_En] -> Drv/2(Step1En)
  Chart/2(Drv_En) -> [DrvST_En]
  [DrvST_Step1_done] -> Chart/4(Drv_done)
  [DrvST_Step1_ini] -> Chart/3(Drv_ini)
  Chart1/4(IfVeSMSbDrvStRclCmdSrv_Val_write) -> IfVeSMSbDrvStRclCmdSrv_Val_write/1
  [DrvST_Step1_done] -> Logical Operator2/2
  [R2LtST_Recovery_done] -> Logical Operator2/1
  Logical Operator2/1 -> Chart1/1(Left_Done), RecoveryLDone/1
  Logical Operator3/1 -> [Recv_L_DoneFailed]
  isLfRecoveryArrivedAtTargetPos/1 -> [Recv_L_DoneOK], Logical Operator3/1

== system ModeAdjust/ModeAdjustRunnable_sys/ModeAdjust/RecoveryR ==
  SecRwRtStPoss : Inport
  SecRwRtStPossV : Inport  Port=2
  SecRwRtStChldLkRsp_R : Inport  Port=3
  Recovery_Mod_Right : Inport  Port=4
  ModeStCalib : Inport  Port=5
  StConfig : Inport  Port=6
  PassStPoss : Inport  Port=7
  PassStPossV : Inport  Port=8
  isRtRecoveryArrivedAtTargetPos : Inport  Port=9
  Enable : EnablePort  StatesWhenEnabling=reset
  Bus Creator2 : BusCreator  Inputs=2
  Bus Selector : BusSelector  OutputSignals=Calib_Drv,Calib_Pass,Calib_2L,Calib_2R,Calib_3L,Calib_3R
  Bus Selector1 : BusSelector  OutputSignals=DrvStConfig,PassStConfig,SecRwLtStConfig,SecRwRtStConfig,ThdRwLtStConfig,ThdRwRtStConfig
  Chart : Stateflow chart  TreatAsAtomicUnit=on
  Chart1 : Stateflow chart  TreatAsAtomicUnit=on
  Logical Operator2 : Logic  AllPortsSameDT=off  OutDataTypeStr=boolean
  Logical Operator3 : Logic  Operator=NOT  AllPortsSameDT=off  OutDataTypeStr=boolean
  Pass : Subsystem
  R2Rt : Subsystem
  VIP_TrigJudg1 : Lib/VIP_TrigJudg  SystemSampleTime=-1
  R2Rt_TrgtPoss : Outport  VectorParamsAs1DForOutWhenUnconnected=on
  IfVeSMSbSecRwRtStRclCmdSrv_Val_writeRec : Outport  Port=2
  isAcsMdFeedBackNew_RecoveryR : Outport  Port=3
  RecoveryRDone : Outport  Port=4
  PassStTrgtPoss : Outport  Port=5  VectorParamsAs1DForOutWhenUnconnected=on
  IfVeSMSuPassStRclCmdSrv_Val_write : Outport  Port=6
  wires:
  [Recovery_R_DoneFailed] -> Bus Creator2/2  "isRfRecoveryDoneFailed"
  [Recovery_R_DoneOK] -> Bus Creator2/1  "isRfRecoveryDoneOK"
  Bus Creator2/1 -> isAcsMdFeedBackNew_RecoveryR/1
  VIP_TrigJudg1/1 -> [EZE_TrigR]
  [Recovery_Mod_Right] -> VIP_TrigJudg1/1
  [ModeStCalib_2R] -> R2Rt/6(ModeStCalib_2R)
  ModeStCalib/1 -> Bus Selector/1
  Bus Selector/4 -> [ModeStCalib_2R]  "<Calib_2R>"
  Bus Selector/6 -> [ModeStCalib_3R]  "<Calib_3R>"
  Bus Selector/1 -> [ModeStCalib_Drv]  "<Calib_Drv>"
  Bus Selector/3 -> [ModeStCalib_2L]  "<Calib_2L>"
  Bus Selector/5 -> [ModeStCalib_3L]  "<Calib_3L>"
  Bus Selector/2 -> [ModeStCalib_Pass]  "<Calib_Pass>"
  Chart1/1(IfVeSMSbSecRwRtStRclCmdSrv_Val_write) -> IfVeSMSbSecRwRtStRclCmdSrv_Val_writeRec/1  "IfVeSMSbSecRwRtStRclCmdSrv_Val_write"
  Chart1/3(Md_R_DoneFailed) -> [Recovery_R_DoneFailed]
  Chart1/2(Md_R_DoneOk) -> [Recovery_R_DoneOK]
  [Recv_R_DoneFailed] -> Chart1/4(Md_R_DoneFailedRaw)
  [Recv_R_DoneOK] -> Chart1/3(Md_R_DoneOkRaw)
  Chart/1(R2Rt_En) -> [R_R2Rt_En]
  [R_R2Rt_En] -> R2Rt/2(Step1En)
  [R2RtST_Recovery_done] -> Chart/2(R2Rt_done)
  [R2RtST_Recovery_ini] -> Chart/1(R2Rt_ini)
  SecRwRtStChldLkRsp_R/1 -> Pass/7(SecRwRtStChldLkRsp_L), R2Rt/5(SecRwRtStChldLkRsp_L)
  SecRwRtStPossV/1 -> R2Rt/4(SecRwRtStPossV)
  SecRwRtStPoss/1 -> R2Rt/3(SecRwRtStPoss)
  R2Rt/3(R2Rt_TrgtPoss) -> R2Rt_TrgtPoss/1
  [EZE_TrigR] -> R2Rt/1(Mode_Trig)
  R2Rt/2(R2RtSt_Recovery_done) -> [R2RtST_Recovery_done]
  R2Rt/1(R2RtSt_Recovery_ini) -> [R2RtST_Recovery_ini]
  Recovery_Mod_Right/1 -> [Recovery_Mod_Right]
  [IfVeSMSbSecRwRtStRclCmdSrv_Val_writeRaw] -> Chart1/2(IfVeSMSbSecRwRtStRclCmdSrv_Val_writeRaw)
  R2Rt/4(IfVeSMSbSecRwRtStRclCmdSrv_Val_writeRaw) -> [IfVeSMSbSecRwRtStRclCmdSrv_Val_writeRaw]
  Bus Selector1/6 -> [ThdRwRtStConfig]  "<ThdRwRtStConfig>"
  Bus Selector1/1 -> [DrvStConfig]  "<DrvStConfig>"
  Bus Selector1/3 -> [SecRwLtStConfig]  "<SecRwLtStConfig>"
  Bus Selector1/4 -> [SecRwRtStConfig]  "<SecRwRtStConfig>"
  StConfig/1 -> Bus Selector1/1
  Bus Selector1/2 -> [PassStConfig]  "<PassStConfig>"
  Bus Selector1/5 -> [ThdRwLtStConfig]  "<ThdRwLtStConfig>"
  [SecRwRtStConfig] -> R2Rt/7(StConfig)
  [PassStConfig] -> Pass/6(StConfig)
  [ModeStCalib_Pass] -> Pass/5(ModeStCalib_Pass)
  [PassST_En_Step1] -> Pass/2(Step1En)
  PassStPossV/1 -> Pass/4(PassStPossV)
  [EZE_TrigR] -> Pass/1(Mode_Trig)
  Pass/4(IfVeSMSuPassStRclCmdSrv_Val_writeRaw) -> [IfVeSMSuPassStRclCmdSrv_Val_writeRaw]
  Pass/3(PassStTrgtPoss) -> PassStTrgtPoss/1
  Pass/1(Pass_Step1_ini) -> [PassST_Step1_ini]
  PassStPoss/1 -> Pass/3(PassStPoss)
  Pass/2(Pass_Step1_done) -> [Pass_Step1_done]
  Chart/2(PassSt_En) -> [PassST_En_Step1]
  [PassST_Step1_ini] -> Chart/3(PassSt_ini)
  [Pass_Step1_done] -> Chart/4(PassSt_done)
  Logical Operator2/1 -> RecoveryRDone/1, Chart1/1(Right_Done)
  [R2RtST_Recovery_done] -> Logical Operator2/1
  [Pass_Step1_done] -> Logical Operator2/2
  [IfVeSMSuPassStRclCmdSrv_Val_writeRaw] -> Chart1/5(IfVeSMSuPassStRclCmdSrv_Val_writeRaw)
  Chart1/4(IfVeSMSuPassStRclCmdSrv_Val_write) -> IfVeSMSuPassStRclCmdSrv_Val_write/1
  Logical Operator3/1 -> [Recv_R_DoneFailed]
  isRtRecoveryArrivedAtTargetPos/1 -> [Recv_R_DoneOK], Logical Operator3/1

== system ModeAdjust/ModeAdjustRunnable_sys/ModeAdjust/RecvyL4s ==
  note: Change Request 179276
      | 复位模式头枕上下移动到第一步，第一步直接控制靠背、头枕上下、腿托系统同时运动，
      | 当腿托系统运动完成后进行头枕前后运动
  SecRwLtStsPoss : Inport
  SecRwLtStPossV : Inport  Port=2
  SecRwRtStChldLkRsp_L : Inport  Port=3
  Recovery_Mod_Left : Inport  Port=4
  ModeStCalib : Inport  Port=5
  StConfig : Inport  Port=6
  SecRwLtStsPoss4s : Inport  Port=7
  SecRwLtStPossV4s : Inport  Port=8
  StConfig4s : Inport  Port=9
  isLfRecoveryArrivedAtTargetPos : Inport  Port=10
  Calib_Recovery4sLAdpt : Inport  Port=11
  Enable : EnablePort  StatesWhenEnabling=reset
  Bus Creator1 : BusCreator  Inputs=2
  Bus Selector : BusSelector  OutputSignals=Calib_Drv,Calib_Pass,Calib_2L,Calib_2R,Calib_3L,Calib_3R,Calib_2L4s,Calib_2R4s
  Bus Selector1 : BusSelector  OutputSignals=DrvStConfig,PassStConfig,SecRwLtStConfig,SecRwRtStConfig,ThdRwLtStConfig,ThdRwRtStConfig
  Bus Selector2 : BusSelector  OutputSignals=SecRwLtStConfig,SecRwRtStConfig
  Bus Selector3 : BusSelector  OutputSignals=IfVeSMSuSecRwLtStBkReclnUpwdDnwdPos_Val_read,IfVeSMSuSecRwLtStFrwdBkwdPos_Val_read,IfVeSMSuSecRwLtStHPassStUpwdDnwdPos_Val_read,IfVeSMSuSecRwLtStLgrstUpwdDnwdPos_Val_read,IfVeSMSuSecRwLtStLtwdRtwdPos_Val_read,IfVeSMSuSecRwLtStArmScrnPos_Val_read
  Bus Selector4 : BusSelector  OutputSignals=IfVeSMSuSecRwLtStBkReclnUpwdDnwdPosV_Val_read,IfVeSMSuSecRwLtStFrwdBkwdPosV_Val_read,IfVeSMSuSecRwLtStHPassStUpwdDnwdPosV_Val_read,IfVeSMSuSecRwLtStLgrstUpwdDnwdPosV_Val_read,IfVeSMSuSecRwLtStLtwdRtwdPosV_Val_read,IfVeSMSuSecRwLtStArmScrnPosV_Val_read
  Bus Selector5 : BusSelector  OutputSignals=IfVeSMSuSecRwLtStLgrstOtwdInwdPos_Val_read,IfVeSMSuRrLtStFtUpwdDnwdPos_Val_read,IfVeSMSuSecRwLtStHdrstFrwdBkwdPos_Val_read
  Bus Selector6 : BusSelector  OutputSignals=IfVeSMSuSecRwLtStLgrstOtwdInwdPosV_Val_read,IfVeSMSuRrLtStFtUpwdDnwdPosV_Val_read
  Chart : Stateflow chart  TreatAsAtomicUnit=on
  Chart1 : Stateflow chart  TreatAsAtomicUnit=on
  Logical Operator : Logic  Inputs=4  AllPortsSameDT=off  OutDataTypeStr=boolean
  Logical Operator1 : Logic  Operator=NOT  AllPortsSameDT=off  OutDataTypeStr=boolean
  Logical Operator2 : Logic  Inputs=3  AllPortsSameDT=off  OutDataTypeStr=boolean
  Logical Operator3 : Logic  Operator=OR  AllPortsSameDT=off  OutDataTypeStr=boolean
  PA_KeSMSuSecRwStFtrstUpwdDnwdPosDelta_Val : Constant  Value=KeSMSuSecRwStFtrstUpwdDnwdPosDelta_Val
  PA_KeSMSuSecRwStLegrestInOutPosDelta_Val : Constant  Value=KeSMSuSecRwStLegrestInOutPosDelta_Val
  PA_KeSMSw4SSecRwLtStLgrstOtwdInwdClosePos1_Val : Constant  Value=KeSMSw4SSecRwLtStLgrstOtwdInwdClosePos1_Val
  PA_KeSMSw4SSecRwLtStLgrstUpwdDnwdClosePos1_Val : Constant  Value=KeSMSw4SSecRwLtStLgrstUpwdDnwdClosePos1_Val
  PA_KeSMSw4SSecRwLtStLgrstUpwdDnwdClosePos2_Val : Constant  Value=KeSMSw4SSecRwLtStLgrstUpwdDnwdClosePos2_Val
  R2Lt : Subsystem
  VIP_TrigJudg : Lib/VIP_TrigJudg  SystemSampleTime=-1
  R2Lt_TrgtPoss : Outport  VectorParamsAs1DForOutWhenUnconnected=on
  IfVeSMSuSecRwLtStRclCmdSrv_Val_writeRec : Outport  Port=2
  isAcsMdFeedBackNew_LyL : Outport  Port=3
  R2Lt_TrgtPoss_2 : Outport  Port=4  VectorParamsAs1DForOutWhenUnconnected=on
  wires:
  R2Lt/4(IfVeSMSuSecRwLtStRclCmdSrv_Val_writeRaw) -> [IfVeSMSuSecRwLtStRclCmdSrv_Val_writeRaw]
  [IfVeSMSuSecRwLtStRclCmdSrv_Val_writeRaw] -> Chart1/2(IfVeSMSuSecRwLtStRclCmdSrv_Val_writeRaw)
  Recovery_Mod_Left/1 -> [Recovery_Mod_Left]
  Logical Operator/1 -> Chart1/1(Left_Done)
  R2Lt/1(R2Lt_Bk_Ini) -> [R2LtST_BkHd_ini]
  [Step1_En] -> R2Lt/2(Step1En)
  VIP_TrigJudg/1 -> [EZE_TrigL]
  [EZE_TrigL] -> R2Lt/1(Mode_Trig)
  R2Lt/3(R2Lt_TrgtPoss) -> R2Lt_TrgtPoss/1
  SecRwLtStsPoss/1 -> [Pos], R2Lt/3(SecRwLtStsPoss)
  SecRwLtStPossV/1 -> [PosV], R2Lt/4(SecRwLtStPossV)
  SecRwRtStChldLkRsp_L/1 -> R2Lt/5(SecRwRtStChldLkRsp_L)
  R2Lt/2(R2Lt_Bk_done) -> [R2LtST_BkHd_done]
  [R2LtST_BkHd_ini] -> Chart/1(R2Lt_ini)
  [R2LtST_BkHd_done] -> Chart/2(R2Lt_done)
  Chart/1(R2Lt_En) -> [Step1_En]
  [Recv_L_DoneOK] -> Chart1/3(Md_L_DoneOkRaw)
  [Recv_L_DoneFailed] -> Chart1/4(Md_L_DoneFailedRaw)
  Chart1/2(Md_L_DoneOk) -> [Ly_L_DoneOK]
  Chart1/3(Md_L_DoneFailed) -> [Ly_L_DoneFailed]
  Chart1/1(IfVeSMSuSecRwLtStRclCmdSrv_Val_write) -> IfVeSMSuSecRwLtStRclCmdSrv_Val_writeRec/1  "IfVeSMSuSecRwLtStRclCmdSrv_Val_write"
  Bus Selector/2 -> [ModeStCalib_Pass]  "<Calib_Pass>"
  Bus Selector/5 -> [ModeStCalib_3L]  "<Calib_3L>"
  Bus Selector/3 -> [ModeStCalib_2L]  "<Calib_2L>"
  Bus Selector/1 -> [ModeStCalib_Drv]  "<Calib_Drv>"
  Bus Selector/6 -> [ModeStCalib_3R]  "<Calib_3R>"
  Bus Selector/4 -> [ModeStCalib_2R]  "<Calib_2R>"
  ModeStCalib/1 -> Bus Selector/1
  [ModeStCalib_2L4s] -> R2Lt/6(ModeStCalib_2L)
  [Recovery_Mod_Left] -> VIP_TrigJudg/1
  Bus Creator1/1 -> isAcsMdFeedBackNew_LyL/1
  [Ly_L_DoneOK] -> Bus Creator1/1  "isLfRecoveryDoneOK"
  [Ly_L_DoneFailed] -> Bus Creator1/2  "isLfRecoveryDoneFailed"
  Bus Selector1/6 -> [ThdRwRtStConfig]  "<ThdRwRtStConfig>"
  Bus Selector1/1 -> [DrvStConfig]  "<DrvStConfig>"
  Bus Selector1/3 -> [SecRwLtStConfig]  "<SecRwLtStConfig>"
  Bus Selector1/4 -> [SecRwRtStConfig]  "<SecRwRtStConfig>"
  StConfig/1 -> Bus Selector1/1
  Bus Selector1/2 -> [PassStConfig]  "<PassStConfig>"
  Bus Selector1/5 -> [ThdRwLtStConfig]  "<ThdRwLtStConfig>"
  [SecRwLtStConfig] -> R2Lt/7(StConfig)
  Bus Selector/8 -> [ModeStCalib_2R4s]  "<Calib_2R4s>"
  Bus Selector/7 -> [ModeStCalib_2L4s]  "<Calib_2L4s>"
  SecRwLtStsPoss4s/1 -> [Pos4s], R2Lt/8(SecRwLtStsPoss4s)
  SecRwLtStPossV4s/1 -> [PosV4s], R2Lt/9(SecRwLtStPossV4s)
  StConfig4s/1 -> Bus Selector2/1
  Bus Selector2/1 -> [SecRwLtStConfig4s]  "<SecRwLtStConfig>"
  Bus Selector2/2 -> [SecRwRtStConfig4s]  "<SecRwRtStConfig>"
  [SecRwLtStConfig4s] -> R2Lt/10(StConfig4s)
  [PosV] -> Bus Selector4/1
  Bus Selector4/6 -> [R2LtStArmScrnPosV]  "<IfVeSMSuSecRwLtStArmScrnPosV_Val_read>"
  Bus Selector3/6 -> [R2LtStArmScrnPos]  "<IfVeSMSuSecRwLtStArmScrnPos_Val_read>"
  Bus Selector4/5 -> [SecRwLtStLtwdRtwdPosV]  "<IfVeSMSuSecRwLtStLtwdRtwdPosV_Val_read>"
  Bus Selector3/4 -> [SecRwLtStLgrstUpwdDnwdPos]  "<IfVeSMSuSecRwLtStLgrstUpwdDnwdPos_Val_read>"
  Bus Selector3/1 -> [SecRwLtStBkReclnUpwdDnwdPos]  "<IfVeSMSuSecRwLtStBkReclnUpwdDnwdPos_Val_read>"
  Bus Selector3/2 -> [SecRwLtStFrwdBkwdPos]  "<IfVeSMSuSecRwLtStFrwdBkwdPos_Val_read>"
  Bus Selector4/2 -> [SecRwLtStFrwdBkwdPosV]  "<IfVeSMSuSecRwLtStFrwdBkwdPosV_Val_read>"
  Bus Selector4/4 -> [SecRwLtStLgrstUpwdDnwdPosV]  "<IfVeSMSuSecRwLtStLgrstUpwdDnwdPosV_Val_read>"
  Bus Selector3/3 -> [SecRwLtStHPassStUpwdDnwdPos]  "<IfVeSMSuSecRwLtStHPassStUpwdDnwdPos_Val_read>"
  [Pos] -> Bus Selector3/1
  Bus Selector3/5 -> [SecRwLtStLtwdRtwdPos]  "<IfVeSMSuSecRwLtStLtwdRtwdPos_Val_read>"
  Bus Selector4/3 -> [SecRwLtStHPassStUpwdDnwdPosV]  "<IfVeSMSuSecRwLtStHPassStUpwdDnwdPosV_Val_read>"
  Bus Selector4/1 -> [SecRwLtStBkReclnUpwdDnwdPosV]  "<IfVeSMSuSecRwLtStBkReclnUpwdDnwdPosV_Val_read>"
  Bus Selector6/1 -> [SecRwLtStLgrstOtwdInwdPosV]  "<IfVeSMSuSecRwLtStLgrstOtwdInwdPosV_Val_read>"
  [Pos4s] -> Bus Selector5/1
  Bus Selector6/2 -> [RrLtStFtUpwdDnwdPosV]  "<IfVeSMSuRrLtStFtUpwdDnwdPosV_Val_read>"
  [PosV4s] -> Bus Selector6/1
  Bus Selector5/1 -> [SecRwLtStLgrstOtwdInwdPos]  "<IfVeSMSuSecRwLtStLgrstOtwdInwdPos_Val_read>"
  Bus Selector5/2 -> [RrLtStFtUpwdDnwdPos]  "<IfVeSMSuRrLtStFtUpwdDnwdPos_Val_read>"
  [SecRwLtStLgrstUpwdDnwdPos] -> Chart/3(downpos)
  [lgrstStep1_done] -> Chart/9(Step1done)
  [lgrstStep1_ini] -> Chart/12(Step1_ini)
  [lgrstStep2_ini] -> Chart/13(Step2_ini)
  [lgrstStep3_ini] -> Chart/14(Step3_ini)
  [lgrstStep2_done] -> Chart/10(Step2done)
  Chart/2(StepEn_LgrstStep1) -> [StepEn_LgrstStep1]
  Chart/3(StepEn_LgrstStep2) -> [StepEn_LgrstStep2]
  Chart/4(StepEn_LgrstStep3) -> [StepEn_LgrstStep3]
  R2Lt/11(R2Lt_TrgtPoss_2) -> R2Lt_TrgtPoss_2/1
  [lgrstStep3_done] -> Chart/11(Step3done)
  PA_KeSMSw4SSecRwLtStLgrstOtwdInwdClosePos1_Val/1 -> [CloseOtwdPos1]
  PA_KeSMSw4SSecRwLtStLgrstUpwdDnwdClosePos2_Val/1 -> [CloseDnwdPos2]
  PA_KeSMSw4SSecRwLtStLgrstUpwdDnwdClosePos1_Val/1 -> [CloseDnwdPos1]
  [CloseDnwdPos2] -> Chart/7(closedownpos2)
  [CloseDnwdPos1] -> Chart/6(closedownpos1)
  [CloseOtwdPos1] -> Chart/8(closeOtpos1)
  [RrLtStFtUpwdDnwdPos] -> Chart/5(Ftpos)
  [SecRwLtStLgrstOtwdInwdPos] -> Chart/4(Otpos)
  [StepEn_LgrstStep1] -> R2Lt/13(StepEn_LgrstStep3)
  [StepEn_LgrstStep3] -> R2Lt/12(StepEn_LgrstStep2)
  [StepEn_LgrstStep2] -> R2Lt/11(StepEn_LgrstStep1)
  PA_KeSMSuSecRwStFtrstUpwdDnwdPosDelta_Val/1 -> [KeSMSuSecRwStFtrstUpwdDnwdPosDelta_Val]
  [KeSMSuSecRwStFtrstUpwdDnwdPosDelta_Val] -> Chart/15(FtposDelta)
  R2Lt/8(lgrstStep1_done) -> [lgrstStep2_done]
  R2Lt/10(lgrstStep3_done) -> [lgrstStep1_done]
  R2Lt/9(lgrstStep2_done) -> [lgrstStep3_done]
  R2Lt/5(lgrstUpwd_ini) -> [lgrstStep2_ini]
  R2Lt/7(lgrstOtwd_ini) -> [lgrstStep1_ini]
  R2Lt/6(lgrstFtUpwd_ini) -> [lgrstStep3_ini]
  Logical Operator1/1 -> [Recv_L_DoneFailed]
  isLfRecoveryArrivedAtTargetPos/1 -> [Recv_L_DoneOK], Logical Operator1/1
  Chart/5(HdUp_En) -> [HdUp_En]
  Chart/6(HdFwd_En) -> [HdFwd_En]
  [HFwd_Done] -> Chart/16(HdFwd_Done)
  [HdUp_Done] -> Chart/17(HdUp_Done)
  Bus Selector5/3 -> [SecRwLtStHdrstFrwdBkwdPos]  "<IfVeSMSuSecRwLtStHdrstFrwdBkwdPos_Val_read>"
  R2Lt/14(R2Lt_HdFwd_Ini) -> [HFwd_ini]
  R2Lt/12(R2Lt_HdUp_Ini) -> [HdUp_ini]
  R2Lt/15(R2Lt_HdFwd_Done) -> [HFwd_Done]
  R2Lt/13(R2Lt_HdUp_Done) -> [HdUp_Done]
  [HdUp_En] -> R2Lt/14(HdUp_En)
  [HdFwd_En] -> R2Lt/15(HdFwd_En)
  PA_KeSMSuSecRwStLegrestInOutPosDelta_Val/1 -> [KeSMSuSecRwStLegrestInOutPosDelta_Val]
  [KeSMSuSecRwStLegrestInOutPosDelta_Val] -> Chart/18(OtposDelta)
  Chart/7(failflg) -> [failflg]
  [lgrstStep3_done] -> Logical Operator2/3
  [lgrstStep2_done] -> Logical Operator2/2
  [lgrstStep1_done] -> Logical Operator2/1
  Logical Operator2/1 -> Logical Operator3/1
  [failflg] -> Logical Operator3/2
  Logical Operator3/1 -> Logical Operator/1
  [HdUp_Done] -> Logical Operator/4
  [HFwd_Done] -> Logical Operator/3
  [R2LtST_BkHd_done] -> Logical Operator/2
  [HdUp_ini] -> Chart/19(HdUp_ini)
  [HFwd_ini] -> Chart/20(HFwd_ini)
  Calib_Recovery4sLAdpt/1 -> R2Lt/16(Calib_Recovery4sLAdpt)
